simulink model "WindFarmType4AverageModel"  (R2024b)
settings: Solver=FixedStepDiscrete  StartTime=0.0  StopTime=5  RelTol=1e-4
PreLoadFcn:
  | Ts=50e-6;
InitFcn:
  | xInitial = WindFarmType4AverageModelInit;
  | Ts=50e-6;
undefined symbols (not defined in the file or in its folder): D1, D11, Delta, DiscIntNeverNeededParam, find_system
libraries: spsSecondOrderFilterLib x54, spsabctodq0Lib x30, spsThreePhaseVIMeasurementLib x26, simulink_extras x24, spsFirstOrderFilterLib x24, spsControlledVoltageSourceLib x18, spsThreePhaseTransformerTwoWindingsLib x14, spsThreePhasePISectionLineLib x14, simulink x12, spsSeriesRLCBranchLib x7, spsThreePhaseSeriesRLCLoadLib x7, spsSynchronousMachinepuStandardLib x7
(part 1 of 14)
settings Model: Creator=The MathWorks, Inc.  LastModifiedBy=prankfarsons
settings SolverCC: AlgebraicLoopSolver=TrustRegion  SolverResetMethod=Robust
settings DataIOCC: LimitDataPoints=on  SaveFormat=StructureWithTime  SaveOutput=off  SaveTime=off  ReturnWorkspaceOutputs=off
settings OptimizationCC: ExpressionDepthLimit=2147483647  InitFltsAndDblsToZero=on  LifeSpan=inf
settings DebuggingCC: UnderspecifiedInitializationDetection=Classic  MergeDetectMultiDrivingBlocksExec=none  SolverPrmCheckMsg=warning  FcnCallInpInsideContextMsg=warning  UnconnectedInputMsg=warning  UnconnectedOutputMsg=warning  UnconnectedLineMsg=warning  StateNameClashWarn=warning  SubsystemReferenceDiagnosticForUnitTest=warning  SFUnexpectedBacktrackingDiag=warning  SFNoUnconditionalDefaultTransitionDiag=warning  SFExecutionAtInitializationDiag=none  ArithmeticOperatorsInVariantConditions=warning
settings HardwareCC: ProdBitPerPointer=32  ProdBitPerSizeT=32  ProdBitPerPtrDiffT=32  ProdLargestAtomicFloat=None  ProdIntDivRoundTo=Undefined  ProdEndianess=Unspecified  ProdWordSize=32  ProdHWDeviceType=32-bit Generic
settings ModelReferenceCC: EnableRefExpFcnMdlSchedulingChecks=on  PropagateSignalLabelsOutOfModel=off
settings SFSimCC: SimUseLocalCustomCode=off  CustomCodeUndefinedFunction=UseInterfaceOnly
settings RTWCC: RTWUseLocalCustomCode=off  GPUComputeCapability=3.5  DLArmComputeVersion=19.05
settings CodeAppCC: StateflowObjectComments=on
settings GRTTargetCC: TargetLangStandard=C89/C90 (ANSI)  CombineOutputUpdateFcns=off  GRTInterface=on
settings ConfigComp: CovMetricSettings=dw  CovSaveCumulativeToWorkspaceVar=on  CovSaveSingleToWorkspaceVar=on  CovExternalEMLEnable=off  CovSFcnEnable=off
settings SimscapeCC: SimscapeNormalizeSystem=off

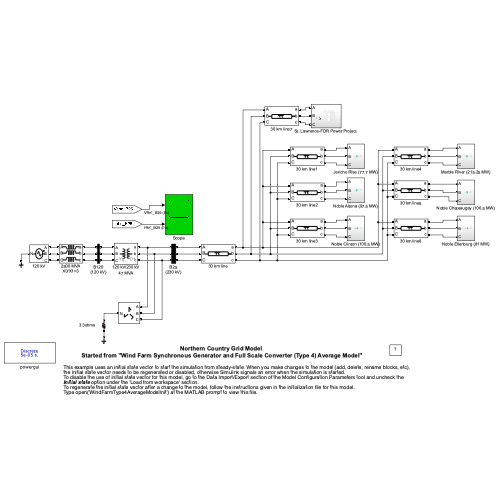
[thumbnail: Simulink's stored preview of the top-level diagram]
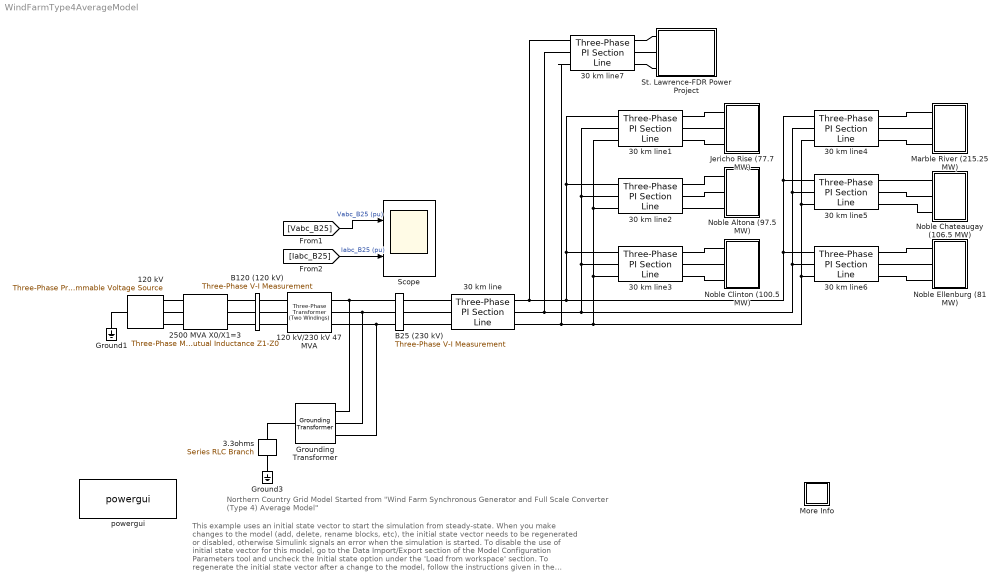
== system WindFarmType4AverageModel ==
  note: Northern Country Grid Model
      | Started from "Wind Farm Synchronous Generator and Full Scale Converter (Type 4) Average Model"
  note: This example uses an initial state vector to start the simulation from steady-state. When you make changes to the model (add, delete, rename blocks, etc),
      | the initial state vector needs to be regenerated or disabled, otherwise Simulink signals an error when the simulation is started.
      | To disable the use of initial state vector for this model, go to the Data Import/Export section of the Model Configuration Parameters tool and uncheck the
      | Initial state option under the 'Load from workspace' section.
      | To regenerate the initial state vector after a change to the model, follow the instructions given in the initialization file for this model.
      | Type open('WindFarmType4AverageModelInit') at the MATLAB prompt to view this file.
  120 kV : spsThreePhaseProgrammableVoltageSourceLib/Three-Phase Programmable Voltage Source  PositiveSequence=[120e3 0 60]  VariationEntity=Amplitude  VariationType=Table of time-amplitude pairs  VariationTypeAlt=Step  VariationStep=-0.2  VariationRate=10  VariationMagnitude=0.3  VariationFrequency=2  VariationTiming=[0.05 0.05+5/60]  VariationPhaseA=off  Amplitudes=[1 0.75 1.0]  TimeValues=[0 0.03 0.13]  HarmonicGeneration=off  HarmonicA=[1 -0.1 0 2]  HarmonicB=[2 0.15 35 2]*0  Timing="[0.1  2]"  BusType=swing  Pref=0  Qref=0  Qmin=-inf  Qmax=inf
  120 kV/230 kV 47 MVA : spsThreePhaseTransformerTwoWindingsLib/Three-Phase Transformer (Two Windings)  Winding1Connection=Yg  Winding2Connection=Delta (D1)  CoreType=Three single-phase transformers  SetSaturation=off  Hysteresis=off  DataFile='basic_model'  SetInitialFlux=off  Measurements=None  UNITS=pu  NominalPower=[47e6 60 ]  Winding1="[ 120e3  0.08/30   0.08 ]"  Winding2="[ 230e3  0.08/30  0.08]"  Rm=500  Lm=500  L0=0.5  Saturation="[ 0,0  ;  0.005,1.2  ;  1.0,1.4 ]"  InitialFluxes=[ 0.8 , -0.8 , 0.7 ]  BreakLoop=off  DiscreteSolver=Trapezoidal iterative  DataType=off  TransfoNumber=0
  2500 MVA X0/X1=3 : spsThreePhaseMutualInductanceZ1Z0Lib/Three-Phase Mutual Inductance Z1-Z0  LConnTagsString=a|b|c  RConnTagsString=A|B|C  PositiveSequence="[0.1  1.0/(2*pi*60)] *120e3^2/2500e6"  ZeroSequence="[0.3  3.0/(2*pi*60)] *120e3^2/2500e6"
      settings: AttributesFormatString=\n
  "3.3ohms " : spsSeriesRLCBranchLib/Series RLC Branch  LConnTagsString=__new0  RConnTagsString=__new0  BranchType=R  Resistance=3.3  Inductance=[]  SetiL0=off  InitialCurrent=0  Capacitance=[]  Setx0=off  InitialVoltage=0  Measurements=None
  30 km line{,1..7} (8 alike) : spsThreePhasePISectionLineLib/Three-Phase PI Section Line  LConnTagsString=a|b|c  RConnTagsString=A|B|C  Length=30  Frequency=60  Resistances=[0.1153 0.413]  Inductances=[1.05e-3 3.32e-3]  Capacitances=[11.33e-009 5.01e-009]
  B120 (120 kV) : spsThreePhaseVIMeasurementLib/Three-Phase V-I Measurement  VoltageMeasurement=no  SetLabelV=off  LabelV=Vabc_B120  Vpu=off  VpuLL=off  CurrentMeasurement=no  SetLabelI=on  LabelI=Iabc_B120  Ipu=off  Pbase=100e6  Vbase=120e3  OutputType=Complex  PhasorSimulation=off  PSBequivalent=0
  B25 (230 kV) : spsThreePhaseVIMeasurementLib/Three-Phase V-I Measurement  VoltageMeasurement=phase-to-ground  SetLabelV=on  LabelV=Vabc_B25  Vpu=on  VpuLL=off  CurrentMeasurement=yes  SetLabelI=on  LabelI=Iabc_B25  Ipu=on  Pbase=77.7e6  Vbase=230e3  OutputType=Complex  PhasorSimulation=off  PSBequivalent=0
  Ground1 : spsGroundLib/Ground  LConnTagsString=a
  Ground3 : spsGroundLib/Ground  LConnTagsString=a
  "Grounding Transformer " : spsGroundingTransformerLib/Grounding Transformer   UNITS=pu  NominalPower="[100e6   60]"  NominalVoltage=25e3  ZeroSequenceImpedance_pu=[0.025 0.75]  MagnetizationBranch_pu=[500 500]  ZeroSequenceImpedance_SI=[0.052083 589.05]  MagnetizationBranch_SI=[1041.7 3.927e+005]  Measurements=None
  Jericho Rise (77.7 MW) : Subsystem
  Marble River (215.25 MW) : Subsystem
  More Info : Subsystem
      settings: OpenFcn="showExample(\"simscapeelectricalsps/WindFarmType4AverageModelExample\")"
      mask Display: disp('?')
  Noble Altona (97.5 MW) : Subsystem
  Noble Chateaugay (106.5 MW) : Subsystem
  Noble Clinton (100.5 MW) : Subsystem
  Noble Ellenburg (81 MW) : Subsystem
  Scope : Scope  NumInputPorts=2
  "St. Lawrence-FDR Power Project " : Subsystem
  powergui : spspowerguiLib/powergui  SimulationMode=Discrete  SampleTime=Ts  frequency=60  Iterations=50  frequencyindice=0  Pbase=100e6  ErrMax=1e-4  UnitsV=kV  UnitsW=MW  buscounter=0  FunctionMessages=off  echomessages=off  EnableUseOfTLC=off  CurrentSourceSwitches=off  DisableSnubberDevices=off  DisableRonSwitches=off  DisableVfSwitches=off  DisplayEquations=off  AutomaticDiscreteSolvers=off  SolverType=Tustin/Backward Euler (TBE)  Interpol=off  ExternalGateDelay=off  methode=off  Ts=0  x0status=blocks  SPID=off  SwTol=0  HookPort=off  NonlinearTolerance=1e-4  nMaxIteration=100  ContinueOnMaxIteration=off  RestoreLinks=warning  ResistiveCurrentMeasurement=off  Frange=[0:2:500]  Ylog=off  Xlog=on  ShowGrid=off  save=off  variable=ZData  structure=0  ZoomFFT=on  StartTime=0.0  cycles=1  DisplayStyle=1  fundamental=60  FreqAxis=off  MaxFrequency=1000  frequencyindicesteady=1  RmsSteady=1  display=off
  wires:
  [Vabc_B25] -> Scope/1  "Vabc_B25 (pu)"
  [Iabc_B25] -> Scope/2  "Iabc_B25 (pu)"
  connections:
  B25 (230 kV)/LConn2 -- 120 kV/230 kV 47 MVA/RConn2 -- "Grounding Transformer "/LConn2
  B25 (230 kV)/LConn3 -- 120 kV/230 kV 47 MVA/RConn3 -- "Grounding Transformer "/LConn3
  B25 (230 kV)/LConn1 -- 120 kV/230 kV 47 MVA/RConn1 -- "Grounding Transformer "/LConn1
  "3.3ohms "/RConn1 -- Ground3/LConn1
  2500 MVA X0/X1=3/RConn1 -- B120 (120 kV)/LConn1
  2500 MVA X0/X1=3/RConn2 -- B120 (120 kV)/LConn2
  2500 MVA X0/X1=3/RConn3 -- B120 (120 kV)/LConn3
  B120 (120 kV)/RConn1 -- 120 kV/230 kV 47 MVA/LConn1
  B120 (120 kV)/RConn2 -- 120 kV/230 kV 47 MVA/LConn2
  B120 (120 kV)/RConn3 -- 120 kV/230 kV 47 MVA/LConn3
  30 km line/LConn1 -- B25 (230 kV)/RConn1
  30 km line/LConn2 -- B25 (230 kV)/RConn2
  30 km line/LConn3 -- B25 (230 kV)/RConn3
  "3.3ohms "/LConn1 -- "Grounding Transformer "/RConn1
  Ground1/LConn1 -- 120 kV/LConn1
  2500 MVA X0/X1=3/LConn1 -- 120 kV/RConn1
  2500 MVA X0/X1=3/LConn2 -- 120 kV/RConn2
  2500 MVA X0/X1=3/LConn3 -- 120 kV/RConn3
  30 km line4/RConn1 -- Marble River (215.25 MW)/LConn1
  30 km line4/RConn2 -- Marble River (215.25 MW)/LConn2
  30 km line4/RConn3 -- Marble River (215.25 MW)/LConn3
  30 km line5/RConn1 -- Noble Chateaugay (106.5 MW)/LConn1
  30 km line5/RConn2 -- Noble Chateaugay (106.5 MW)/LConn2
  30 km line5/RConn3 -- Noble Chateaugay (106.5 MW)/LConn3
  30 km line6/RConn1 -- Noble Ellenburg (81 MW)/LConn1
  30 km line6/RConn2 -- Noble Ellenburg (81 MW)/LConn2
  30 km line6/RConn3 -- Noble Ellenburg (81 MW)/LConn3
  30 km line1/RConn1 -- Jericho Rise (77.7 MW)/LConn1
  30 km line1/RConn2 -- Jericho Rise (77.7 MW)/LConn2
  30 km line1/RConn3 -- Jericho Rise (77.7 MW)/LConn3
  30 km line2/RConn1 -- Noble Altona (97.5 MW)/LConn1
  30 km line2/RConn2 -- Noble Altona (97.5 MW)/LConn2
  30 km line2/RConn3 -- Noble Altona (97.5 MW)/LConn3
  30 km line3/RConn1 -- Noble Clinton (100.5 MW)/LConn1
  30 km line3/RConn2 -- Noble Clinton (100.5 MW)/LConn2
  30 km line3/RConn3 -- Noble Clinton (100.5 MW)/LConn3
  30 km line1/LConn1 -- 30 km line2/LConn1 -- 30 km line3/LConn1 -- 30 km line6/LConn1 -- 30 km line5/LConn1 -- 30 km line4/LConn1 -- 30 km line7/LConn1 -- 30 km line/RConn1
  30 km line1/LConn2 -- 30 km line2/LConn2 -- 30 km line3/LConn2 -- 30 km line6/LConn2 -- 30 km line5/LConn2 -- 30 km line4/LConn2 -- 30 km line7/LConn2 -- 30 km line/RConn2
  30 km line1/LConn3 -- 30 km line2/LConn3 -- 30 km line6/LConn3 -- 30 km line5/LConn3 -- 30 km line4/LConn3 -- 30 km line7/LConn3 -- 30 km line/RConn3 -- 30 km line3/LConn3
  30 km line7/RConn1 -- "St. Lawrence-FDR Power Project "/LConn1
  30 km line7/RConn2 -- "St. Lawrence-FDR Power Project "/LConn2
  30 km line7/RConn3 -- "St. Lawrence-FDR Power Project "/LConn3

== system WindFarmType4AverageModel/Jericho Rise (77.7 MW) ==
  230 kV/34.5 kV 47 MVA : spsThreePhaseTransformerTwoWindingsLib/Three-Phase Transformer (Two Windings)  Winding1Connection=Yg  Winding2Connection=Delta (D1)  CoreType=Three single-phase transformers  SetSaturation=off  Hysteresis=off  DataFile='basic_model'  SetInitialFlux=off  Measurements=None  UNITS=pu  NominalPower=[47e6 60 ]  Winding1="[ 230e3  0.08/30   0.08 ]"  Winding2="[34.5e3  0.08/30  0.08]"  Rm=500  Lm=500  L0=0.5  Saturation="[ 0,0  ;  0.005,1.2  ;  1.0,1.4 ]"  InitialFluxes=[ 0.8 , -0.8 , 0.7 ]  BreakLoop=off  DiscreteSolver=Trapezoidal iterative  DataType=off  TransfoNumber=0
  34.5 kV/ 690V 5*2.5 MVA : spsThreePhaseTransformerTwoWindingsLib/Three-Phase Transformer (Two Windings)  Winding1Connection=Delta (D11)  Winding2Connection=Yg  CoreType=Three single-phase transformers  SetSaturation=off  Hysteresis=off  DataFile='hysteresis'  SetInitialFlux=off  Measurements=None  UNITS=pu  NominalPower="[2.5e6*5  60]"  Winding1=[34.5e3 , 0.025/30 , 0.025]  Winding2=[690, 0.025/30 , 0.025]  Rm=500  Lm=inf  L0=0.5  Saturation=[ 0,0 ; 0.0024,1.2 ; 1.0,1.52 ]  InitialFluxes=[ 0.8 , -0.8 , 0.7 ]  BreakLoop=off  DiscreteSolver=Trapezoidal iterative  DataType=off  TransfoNumber=0
  5 km line : spsThreePhasePISectionLineLib/Three-Phase PI Section Line  LConnTagsString=a|b|c  RConnTagsString=A|B|C  Length=5  Frequency=60  Resistances=[0.1153 0.413]  Inductances=[1.05e-3 3.32e-3]  Capacitances=[11.33e-009 5.01e-009]
  B1 (690 V) : spsThreePhaseVIMeasurementLib/Three-Phase V-I Measurement  VoltageMeasurement=phase-to-ground  SetLabelV=on  LabelV=Vabc_B1  Vpu=on  VpuLL=off  CurrentMeasurement=yes  SetLabelI=on  LabelI=Iabc_B1  Ipu=on  Pbase=37*2.1e6/0.9  Vbase=690  OutputType=Complex  PhasorSimulation=off  PSBequivalent=0
  Bus Selector : BusSelector  OutputSignals=Vdc_V,wr_pu,PQ_pu.P_pu,PQ_pu.Q_pu
  Constant : Constant  Value=15
  Constant1 : Constant  Value=0
  Demux : Demux  Outputs=2
  MW : Gain  Gain=37*2.1/0.9  SaturateOnIntegerOverflow=on  OutDataTypeStr=Inherit: Same as input  ParamDataTypeStr=Inherit: Same as input
  Mux : Mux  Inputs=2
  Wind Farm : Subsystem  LoadFcn=%find_system(gcs,'FollowLinks', 'on', 'LookUnderMasks', 'all');  mask(Wind Turbine: Model 7){Nb_wt=37, ShowParameters=Generator data for 1 wind turbine, nom=[2.1e6/0.9 690 60], Reactances=[ 1.305, 0.296, 0.252, 0.474,  0.243,  0.18 ], Time_constants=[  4.49  0.0681  0.0513  ], Resistance=0.006, mec=[0.62 0.01 1], init=[ 0  0  0  0  0  0  0  0  1 ], Vnom=575, Imax_grid_conv=1.1, RL_grid=[ 0.15 0.15/50], C_var_filter1=150e3, Vdc_nom=1100, C_DClink1=90000e-6, L_R_Boost=[0.0012     5e-3], Pmec1=2e6, wind_speed_CpMax=11, wind0=11, DisplayTurbChar=off, H_WT=4.32, Ksh=0.3, D_mutual=1.5, w_wt0=1, torque0=1, Kdc=[1.1   27.5], Ki_var_reg=0.05, Ki_volt_reg=2, Kgrid_side_cur_reg=[1  50], Kspeed=[5 1], Kboost_cur_reg=[0.025 100], Kp_pitch=15, Kcompensation=[1.5  6], Kfield=[10  20], pitch_max=27, pitch_rate=10, Ts=Ts}
      mask prompts: Nb_wt "Number of wind turbines:"; ShowParameters "Display:"; nom "Nom. power, L-L volt. and freq.: [Pn (VA), Vn (Vrms), fn (Hz)]"; Reactances "Reactances [Xd Xd' Xd'' Xq Xq'' Xl] (p.u.):"; Time_constants "Time constants [Tdo' Tdo'' Tq''] (s):"; Resistance "Resistance Rs (p.u.):"; mec "Inertia constant, friction factor, and pairs of poles: [ H(s)  F(p.u.)  p ]"; init "Initial conditions: [dw(%) th(deg) ia,ib,ic(pu) pha,phb,phc(deg) Vf(pu)]:"; Vnom "Grid-side converter nominal AC voltage (V):"; Imax_grid_conv "Grid-side converter maximum AC current (pu based on generator power and converter nominal AC voltage):"; RL_grid "Grid-side coupling inductor [ L(pu) R(pu),pu based on generator power and converter nominal AC voltage] :"; C_var_filter1 "Line filter capacitor (Q=50) (var):"; Vdc_nom "Nominal DC bus voltage (V)"; C_DClink1 "DC bus capacitor (F):"; L_R_Boost "Boost converter inductance [L(H) R(ohm)]:"; Pmec1 "Nominal mechanical output power (W):"; wind_speed_CpMax "Wind speed at nominal speed and at Cp max (must be between 6 m/s and 30 m/s) (m/s):"; wind0 "Initial wind speed (m/s):"; DisplayTurbChar "Display wind turbine power characteristics:"; H_WT "Wind turbine inertia constant H (s):"; Ksh "Shaft spring constant refer to high-speed shaft (pu of nominal mechanical torque/rad):"; D_mutual "Shaft mutual damping (pu of nominal mechanical torque/pu dw):"; w_wt0 "Turbine initial speed (pu of nominal speed):"; torque0 "Initial output torque (pu of nominal mechanical torque):"; Kdc "DC bus voltage regulator gains [Kp Ki]:"; Ki_var_reg "Grid-side converter var regulator gain [ Ki]:"; Ki_volt_reg "Grid-side converter voltage regulator gain [ Ki]:"; Kgrid_side_cur_reg "Grid-side converter current regulator gains [Kp Ki]:"; Kspeed "Speed regulator gains [Kp Ki]:"; Kboost_cur_reg "Boost inductor current regulator gains [Kp Ki]:"; Kp_pitch "Pitch controller gain [Kp]:"; Kcompensation "Pitch compensation gains [Kp Ki]:"; Kfield "Field excitation gains [Kp Ki]:"; pitch_max "Maximum pitch angle (deg):"; pitch_rate "Maximum rate of change of pitch angle (deg/s)"; Ts "Sample time (s):"
      mask help: This block implements a model of a variable speed pitch controlled wind turbine using a synchronous generator.
      mask init:
      | %Generator data
      | Pnom=nom(1)*Nb_wt;
      | Vnom_gen=nom(2);
      | Fnom=nom(3);
      | Xd=Reactances(1);
      | Xd1=Reactances(2);
      | Xd2=Reactances(3);
      | Xq=Reactances(4);
      | Xq2=Reactances(5);
      | Xl=Reactances(6);
      | Tdo1=Time_constants(1);
      | Tdo2=Time_constants(2);
      | Tq2=Time_constants(3);
      | H=mec(1);
      | F=mec(2);
      | p=mec(3);
      | 
      | % Converters data
      | L_RL=RL_grid(1);
      | R_RL=RL_grid(2);
      | L_Boost=L_R_Boost(1)/Nb_wt;
      | R_Boost=L_R_Boost(2)/Nb_wt;
      | Q_filter=50;
      | C_DClink=C_DClink1*Nb_wt;
      | C_var_filter=C_var_filter1*Nb_wt;
      | 
      | % Controller data
      | Freq_filter=10000;   %Hz
      | Zeta_filter=0.707;
      | Kp_dc=Kdc(1);
      | Ki_dc=Kdc(2);
      | Kp_grid_side_cur_reg=Kgrid_side_cur_reg(1);
      | Ki_grid_side_cur_reg=Kgrid_side_cur_reg(2);
      | Kp_speed=Kspeed(1);
      | Ki_speed=Kspeed(2);
      | Kp_boost_cur_reg=Kboost_cur_reg(1);
      | Ki_boost_cur_reg=Kboost_cur_reg(2);
      | Kp_compensation=Kcompensation(1);
      | Ki_compensation=Kcompensation(2);
      | Kp_field=Kfield(1);
      | Ki_field=Kfield(2);
      | Mod_index_max=1.1;
      | T_speed=5;      %Speed reference time constant (s)
      | Iq_ref_limit_time_constant=0.3; %(s)
      | Current_reg_output_limit=1.1;   %(pu)
      | Var_reg_output_hi_limit=1.1;    %(pu)
      | Var_reg_output_low_limit=0.9;   %(pu)
      | Pitch_time_constant=0.01;       %(s)
      | Vf_limit=10;    %Field voltage limit (pu)
      | Flux_meas_time_constant=1*(1/Fnom); %(s)
      | Ts_snub=50e-6;  %Sample time to compute snubber resistance
      | 
      | 
      | % Turbine data
      | Pmec=Pmec1*Nb_wt;
      | c1 = 0.6450;
      | c2 = 116;
      | c3 = .4;
      | c4 = 5;
      | c5 = 21;
      | c6 = .00912;  % Set Pmin in stall condition (does not vary with wind_speed_Pmax)
      | c7 = .08;
      | c8 = .035;
      | theta=0;
      | CpMax=.5;
      | lambda_CpMax=9.9495;
      | 
      | c1_c8=[c1 c2 c3 c4 c5 c6 c7 c8];
      |   
      | 
      | %   Cp = c1*(c6*lambda + (-c4 - c3*(2.5 + theta) + c2*(1/(lambda + ...
      | %   c7*(2.5 + theta)) - c8/(1 + (2.5 + theta)^3)))/exp(c5*(1/(lambda + ...
      | %   c7*(2.5 + theta)) - c8/(1 + (2.5 + theta)^3))))
      | 
      | 
      |         %%%%%%%%%%%%%%%%%%%%%%%%%%%%%%%%%%%%%%%%%%%%%%%%%%%%%%%%%%%%%%%%%%%%%%%%%%%
      |         % Operation at Cp max
      |         %%%%%%%%%%%%%%%%%%%%%%%%%%%%%%%%%%%%%%%%%%%%%%%%%%%%%%%%%%%%%%%%%%%%%%%%%%%
      |         
      |         rated_omegar=1;
      |         omegar = rated_omegar;
      |         
      |         % Enforce boundaries on wind speed
      |         % A warning could be displayed
      |         if wind_speed_CpMax < 6
      |             wind_speed_CpMax=6;
      |             disp('Warning: Wind speed at nominal speed and at Cp max has been set to 6 m/s')
      |         end
      |         if wind_speed_CpMax > 30
      |             wind_speed_CpMax=30;
      |             disp('Warning: Wind speed at nominal speed and at Cp max has been set to 30 m/s')
      |         end
      | 
      |         K1=lambda_CpMax/omegar*wind_speed_CpMax;
      |         
      |         % Calculation of K2 needed to get P equal to the requested value at
      |         % Cp max for the requested wind speed
      |         
      |         Prated=Pmec;
      |         P_rated_omegar_theta_zero=0.75;
      |         
      |         K2 = P_rated_omegar_theta_zero*Prated/(wind_speed_CpMax^3*CpMax);
      |         
      |         K1_K2=[K1 K2];
      |         
      |         %%%%%%%%%%%%%%%%%%%%%%%%%%%%%%%%%%%%%%%%%%%%%%%%%%%%%%%%%%%%%%%%%%%%%%%%%%%
      |         % End of calculation for operation at Cp max
      |         %%%%%%%%%%%%%%%%%%%%%%%%%%%%%%%%%%%%%%%%%%%%%%%%%%%%%%%%%%%%%%%%%%%%%%%%%%%
      |         
      | 
      | %%%%%%%%%%%%%%%%%%%%%%%%%%%%%%%%%%%%%%%%%%%%%%%%%%%%%%%%%%%%%%%%%%%%%%%%%%%
      | % Plot turbine characteristics
      | %%%%%%%%%%%%%%%%%%%%%%%%%%%%%%%%%%%%%%%%%%%%%%%%%%%%%%%%%%%%%%%%%%%%%%%%%%% 
      | 
      | DisplayTurbChar=get_param(gcb,'DisplayTurbChar');
      | if strcmp(DisplayTurbChar,'on')
      |     vect_theta = 0:2:30;
      |     
      |     vect_lambda = 1:0.2:30;
      |     
      |     clear Cp;
      |     
      |     for i=1:length(vect_theta)
      |      for j=1:length(vect_lambda)
      |                 Cp(i,j) = c1*(c6*vect_lambda(j) + (-c4 - c3*(2.5 + vect_theta(i)) + c2*(1/(vect_lambda(j) + ...
      |                 c7*(2.5 + vect_theta(i))) - c8/(1 + (2.5 + vect_theta(i))^3)))/exp(c5*(1/(vect_lambda(j) + ...
      |                 c7*(2.5 + vect_theta(i))) - c8/(1 + (2.5 + vect_theta(i))^3))));
      |      end
      |     end
      | 
      |     figure(1);
      |     clf;
      |     hold on;
      | 
      |     plot(vect_lambda, Cp);
      |     axis([0, 25, 0, .6]);
      |     title('Wind Turbine Cp Characteristic (pitch angle increases by step of 2 deg.)');
      |     ylabel('Cp');
      |     set(gca,'ytick',[0 .1 .2 .3 .4 .5 .6]);
      |     xlabel('Lambda');
      |     grid on;
      |     text(10.1,0.51,'Pitch angle 0 degree');
      | 
      |     hold off
      |     
      |     % Plot of the wind turbine mechanical power output (pu) lambda and Cp
      |     % characteristics against wind speed (m/s) for a range of theta.
      |     
      |     wind_speed_range = [1,.2,30];
      |     vect_wind_speed = 1:0.2:30;
      |     
      |     clear lambda;
      |     clear Cp;
      |     clear P;
      | 
      |     for i=1:length(vect_theta)
      |         for j=1:length(vect_wind_speed)
      |             lambda(i,j) = K1*omegar/vect_wind_speed(j);
      |             Cp(i,j) = c1*(c6*lambda(i,j) + (-c4 - c3*(2.5 + vect_theta(i)) + c2*(1/(lambda(i,j) + ...
      |             c7*(2.5 + vect_theta(i))) - c8/(1 + (2.5 + vect_theta(i))^3)))/exp(c5*(1/(lambda(i,j) + ...
      |             c7*(2.5 + vect_theta(i))) - c8/(1 + (2.5 + vect_theta(i))^3))));
      |             P(i,j) = K2/Prated*vect_wind_speed(j)^3*Cp(i,j);
      |         end
      |     end
      |     
      |     
      |     figure(2);
      |     clf;
      |     hold on
      |     
      |     subplot(3,1,1);
      |     plot(vect_wind_speed, P);
      |     axis([0, 35, 0, 1.5]);
      |     title('Wind Turbine Characteristics (w = 1 pu, pitch angle increases by step of 2 deg.)');
      |     ylabel('P (pu)');
      |     set(gca,'ytick',0:.5:4);
      |     grid on;
      |     
      |     subplot(3,1,2);
      |     plot(vect_wind_speed, lambda);
      |     axis([0, 35, 0, 20]);
      |     ylabel('Lambda');
      |     grid on;
      |     
      |     subplot(3,1,3)
      |     plot(vect_wind_speed, Cp);
      |     axis([0, 35, 0, .6]);
      |     xlabel('Wind Speed (m/s)');
      |     ylabel('Cp');
      |     set(gca,'ytick',[0 .1 .2 .3 .4 .5 .6]);
      |     grid on;
      | 
      |     hold off
      |     set_param(gcb,'DisplayTurbChar','off')
      |     
      | end
      mask TypeOptions ShowParameters: Generator data for 1 wind turbine | Converters data for 1 wind turbine | Turbine data for 1 wind turbine | Drive train data for 1 wind turbine | Control parameters for 1 wind turbine
      mask Callback ShowParameters:
      | BlockName=getfullname(gcb);
      | %
      | Param_Show=get_param(BlockName,'ShowParameters');
      | Param_DisplayTurbChar=get_param(BlockName,'DisplayTurbChar');
      | 
      | p_mask{3}='off';p_mask{4}='off';p_mask{5}='off';
      | p_mask{6}='off';p_mask{7}='off';p_mask{8}='off';p_mask{9}='off';
      | p_mask{10}='off';p_mask{11}='off';p_mask{12}='off';p_mask{13}='off';
      | p_mask{14}='off';p_mask{15}='off';p_mask{16}='off';p_mask{17}='off';
      | p_mask{18}='off';p_mask{19}='off';p_mask{20}='off';p_mask{21}='off';
      | p_mask{22}='off';p_mask{23}='off';p_mask{24}='off';p_mask{25}='off';
      | p_mask{26}='off';p_mask{27}='off';p_mask{28}='off';p_mask{29}='off';
      | p_mask{30}='off';p_mask{31}='off';p_mask{32}='off';p_mask{33}='off';
      | p_mask{34}='off';p_mask{35}='off';
      | 
      | switch Param_Show
      | 	case 'Generator data for 1 wind turbine'
      | 		p_mask{3}='on';p_mask{4}='on';p_mask{5}='on';
      |         p_mask{6}='on';p_mask{7}='on';p_mask{8}='on';
      |     case 'Converters data for 1 wind turbine'
      | 		p_mask{9}='on';p_mask{10}='on';p_mask{11}='on';
      |         p_mask{12}='on';p_mask{13}='on';p_mask{14}='on';p_mask{15}='on';
      | 	case 'Turbine data for 1 wind turbine'
      | 		p_mask{16}='on';p_mask{17}='on';p_mask{18}='on';p_mask{19}='on';
      |     case 'Drive train data for 1 wind turbine'
      |         p_mask{20}='on';p_mask{21}='on';p_mask{22}='on';p_mask{23}='on';
      |         p_mask{24}='on';
      |     case 'Control parameters for 1 wind turbine'
      |         p_mask{25}='on';p_mask{26}='on';p_mask{27}='on';
      |         p_mask{28}='on';p_mask{29}='on';p_mask{30}='on';p_mask{31}='on';
      |         p_mask{32}='on';p_mask{33}='on';p_mask{34}='on';p_mask{35}='on';
      | end
      | 
      | ParVisible={'on','on',p_mask{3},p_mask{4},p_mask{5},p_mask{6},...
      |     p_mask{7},p_mask{8},p_mask{9},p_mask{10},p_mask{11},p_mask{12},...
      |     p_mask{13},p_mask{14},p_mask{15},p_mask{16},p_mask{17},p_mask{18},...
      |     p_mask{19},p_mask{20},p_mask{21},p_mask{22},p_mask{23},p_mask{24},...
      |     p_mask{25},p_mask{26},p_mask{27},p_mask{28},p_mask{29},p_mask{30},...
      |     p_mask{31},p_mask{32},p_mask{33},p_mask{34},p_mask{35},'on'};
      | %
      | set_param(BlockName,'MaskVisibilities',ParVisible);
      | set_param(BlockName,'DisplayTurbChar',Param_DisplayTurbChar);
      mask Display: disp(' ');
  Wind Farm Scope : Scope  NumInputPorts=6
  A : PMIOPort  Side=Left
  B : PMIOPort  Port=2  Side=Left
  C : PMIOPort  Port=3  Side=Left
  wires:
  Constant1/1 -> Wind Farm/2(Qref_pu)
  [Vabc_B1] -> Wind Farm Scope/1  "Vabc_B575 (pu)"
  Demux/1 -> Wind Farm Scope/5  "P (MW)"
  Bus Selector/1 -> Wind Farm Scope/3  "<Vdc_V>"
  Demux/2 -> Wind Farm Scope/6  "Q (Mvar)"
  Mux/1 -> MW/1
  Bus Selector/2 -> Wind Farm Scope/4  "<wr_pu>"
  Wind Farm/1(m) -> Bus Selector/1
  Bus Selector/3 -> Mux/1  "<P_pu>"
  Bus Selector/4 -> Mux/2  "<Q_pu>"
  MW/1 -> Demux/1
  [Iabc_B1] -> Wind Farm Scope/2  "Iabc_B575 (pu)"
  Constant/1 -> Wind Farm/1("Wind (m/s) ")
  connections:
  B1 (690 V)/LConn2 -- 34.5 kV/ 690V 5*2.5 MVA/RConn2
  B1 (690 V)/RConn1 -- Wind Farm/LConn1
  B1 (690 V)/LConn1 -- 34.5 kV/ 690V 5*2.5 MVA/RConn1
  B1 (690 V)/LConn3 -- 34.5 kV/ 690V 5*2.5 MVA/RConn3
  B1 (690 V)/RConn3 -- Wind Farm/LConn3
  Wind Farm/LConn2 -- B1 (690 V)/RConn2
  5 km line/RConn1 -- 34.5 kV/ 690V 5*2.5 MVA/LConn1
  5 km line/RConn2 -- 34.5 kV/ 690V 5*2.5 MVA/LConn2
  5 km line/LConn1 -- 230 kV/34.5 kV 47 MVA/RConn1
  5 km line/LConn2 -- 230 kV/34.5 kV 47 MVA/RConn2
  5 km line/LConn3 -- 230 kV/34.5 kV 47 MVA/RConn3
  A/RConn1 -- 230 kV/34.5 kV 47 MVA/LConn1
  B/RConn1 -- 230 kV/34.5 kV 47 MVA/LConn2
  C/RConn1 -- 230 kV/34.5 kV 47 MVA/LConn3
  5 km line/RConn3 -- 34.5 kV/ 690V 5*2.5 MVA/LConn3

== system WindFarmType4AverageModel/Marble River (215.25 MW) ==
  230 kV/34.5 kV 47 MVA : spsThreePhaseTransformerTwoWindingsLib/Three-Phase Transformer (Two Windings)  Winding1Connection=Yg  Winding2Connection=Delta (D1)  CoreType=Three single-phase transformers  SetSaturation=off  Hysteresis=off  DataFile='basic_model'  SetInitialFlux=off  Measurements=None  UNITS=pu  NominalPower=[47e6 60 ]  Winding1="[ 230e3  0.08/30   0.08 ]"  Winding2="[34.5e3  0.08/30  0.08]"  Rm=500  Lm=500  L0=0.5  Saturation="[ 0,0  ;  0.005,1.2  ;  1.0,1.4 ]"  InitialFluxes=[ 0.8 , -0.8 , 0.7 ]  BreakLoop=off  DiscreteSolver=Trapezoidal iterative  DataType=off  TransfoNumber=0
  34.5 kV/ 690V 5*2.5 MVA : spsThreePhaseTransformerTwoWindingsLib/Three-Phase Transformer (Two Windings)  Winding1Connection=Delta (D11)  Winding2Connection=Yg  CoreType=Three single-phase transformers  SetSaturation=off  Hysteresis=off  DataFile='hysteresis'  SetInitialFlux=off  Measurements=None  UNITS=pu  NominalPower="[2.5e6*5  60]"  Winding1=[34.5e3 , 0.025/30 , 0.025]  Winding2=[690, 0.025/30 , 0.025]  Rm=500  Lm=inf  L0=0.5  Saturation=[ 0,0 ; 0.0024,1.2 ; 1.0,1.52 ]  InitialFluxes=[ 0.8 , -0.8 , 0.7 ]  BreakLoop=off  DiscreteSolver=Trapezoidal iterative  DataType=off  TransfoNumber=0
  5 km line : spsThreePhasePISectionLineLib/Three-Phase PI Section Line  LConnTagsString=a|b|c  RConnTagsString=A|B|C  Length=5  Frequency=60  Resistances=[0.1153 0.413]  Inductances=[1.05e-3 3.32e-3]  Capacitances=[11.33e-009 5.01e-009]
  B2 (690 V) : spsThreePhaseVIMeasurementLib/Three-Phase V-I Measurement  VoltageMeasurement=phase-to-ground  SetLabelV=on  LabelV=Vabc_B2  Vpu=on  VpuLL=off  CurrentMeasurement=yes  SetLabelI=on  LabelI=Iabc_B2  Ipu=on  Pbase=5*2e6/0.9  Vbase=690  OutputType=Complex  PhasorSimulation=off  PSBequivalent=0
  Bus Selector : BusSelector  OutputSignals=Vdc_V,wr_pu,PQ_pu.P_pu,PQ_pu.Q_pu
  Constant : Constant  Value=15
  Constant1 : Constant  Value=0
  Demux : Demux  Outputs=2
  MW : Gain  Gain=70*3.075/0.9  SaturateOnIntegerOverflow=on  OutDataTypeStr=Inherit: Same as input  ParamDataTypeStr=Inherit: Same as input
  Mux : Mux  Inputs=2
  Wind Farm : Subsystem  LoadFcn=%find_system(gcs,'FollowLinks', 'on', 'LookUnderMasks', 'all');  mask(Wind Turbine: Model 7){Nb_wt=70, ShowParameters=Generator data for 1 wind turbine, nom=[3.075e6/0.9 690 60], Reactances=[ 1.305, 0.296, 0.252, 0.474,  0.243,  0.18 ], Time_constants=[  4.49  0.0681  0.0513  ], Resistance=0.006, mec=[0.62 0.01 1], init=[ 0  0  0  0  0  0  0  0  1 ], Vnom=575, Imax_grid_conv=1.1, RL_grid=[ 0.15 0.15/50], C_var_filter1=150e3, Vdc_nom=1100, C_DClink1=90000e-6, L_R_Boost=[0.0012     5e-3], Pmec1=2e6, wind_speed_CpMax=11, wind0=11, DisplayTurbChar=off, H_WT=4.32, Ksh=0.3, D_mutual=1.5, w_wt0=1, torque0=1, Kdc=[1.1   27.5], Ki_var_reg=0.05, Ki_volt_reg=2, Kgrid_side_cur_reg=[1  50], Kspeed=[5 1], Kboost_cur_reg=[0.025 100], Kp_pitch=15, Kcompensation=[1.5  6], Kfield=[10  20], pitch_max=27, pitch_rate=10, Ts=Ts}
      mask prompts: Nb_wt "Number of wind turbines:"; ShowParameters "Display:"; nom "Nom. power, L-L volt. and freq.: [Pn (VA), Vn (Vrms), fn (Hz)]"; Reactances "Reactances [Xd Xd' Xd'' Xq Xq'' Xl] (p.u.):"; Time_constants "Time constants [Tdo' Tdo'' Tq''] (s):"; Resistance "Resistance Rs (p.u.):"; mec "Inertia constant, friction factor, and pairs of poles: [ H(s)  F(p.u.)  p ]"; init "Initial conditions: [dw(%) th(deg) ia,ib,ic(pu) pha,phb,phc(deg) Vf(pu)]:"; Vnom "Grid-side converter nominal AC voltage (V):"; Imax_grid_conv "Grid-side converter maximum AC current (pu based on generator power and converter nominal AC voltage):"; RL_grid "Grid-side coupling inductor [ L(pu) R(pu),pu based on generator power and converter nominal AC voltage] :"; C_var_filter1 "Line filter capacitor (Q=50) (var):"; Vdc_nom "Nominal DC bus voltage (V)"; C_DClink1 "DC bus capacitor (F):"; L_R_Boost "Boost converter inductance [L(H) R(ohm)]:"; Pmec1 "Nominal mechanical output power (W):"; wind_speed_CpMax "Wind speed at nominal speed and at Cp max (must be between 6 m/s and 30 m/s) (m/s):"; wind0 "Initial wind speed (m/s):"; DisplayTurbChar "Display wind turbine power characteristics:"; H_WT "Wind turbine inertia constant H (s):"; Ksh "Shaft spring constant refer to high-speed shaft (pu of nominal mechanical torque/rad):"; D_mutual "Shaft mutual damping (pu of nominal mechanical torque/pu dw):"; w_wt0 "Turbine initial speed (pu of nominal speed):"; torque0 "Initial output torque (pu of nominal mechanical torque):"; Kdc "DC bus voltage regulator gains [Kp Ki]:"; Ki_var_reg "Grid-side converter var regulator gain [ Ki]:"; Ki_volt_reg "Grid-side converter voltage regulator gain [ Ki]:"; Kgrid_side_cur_reg "Grid-side converter current regulator gains [Kp Ki]:"; Kspeed "Speed regulator gains [Kp Ki]:"; Kboost_cur_reg "Boost inductor current regulator gains [Kp Ki]:"; Kp_pitch "Pitch controller gain [Kp]:"; Kcompensation "Pitch compensation gains [Kp Ki]:"; Kfield "Field excitation gains [Kp Ki]:"; pitch_max "Maximum pitch angle (deg):"; pitch_rate "Maximum rate of change of pitch angle (deg/s)"; Ts "Sample time (s):"
      mask help: This block implements a model of a variable speed pitch controlled wind turbine using a synchronous generator.
      mask init: same as WindFarmType4AverageModel/Jericho Rise (77.7 MW)/Wind Farm
      mask TypeOptions ShowParameters: Generator data for 1 wind turbine | Converters data for 1 wind turbine | Turbine data for 1 wind turbine | Drive train data for 1 wind turbine | Control parameters for 1 wind turbine
      mask Callback ShowParameters:
      | BlockName=getfullname(gcb);
      | %
      | Param_Show=get_param(BlockName,'ShowParameters');
      | Param_DisplayTurbChar=get_param(BlockName,'DisplayTurbChar');
      | 
      | p_mask{3}='off';p_mask{4}='off';p_mask{5}='off';
      | p_mask{6}='off';p_mask{7}='off';p_mask{8}='off';p_mask{9}='off';
      | p_mask{10}='off';p_mask{11}='off';p_mask{12}='off';p_mask{13}='off';
      | p_mask{14}='off';p_mask{15}='off';p_mask{16}='off';p_mask{17}='off';
      | p_mask{18}='off';p_mask{19}='off';p_mask{20}='off';p_mask{21}='off';
      | p_mask{22}='off';p_mask{23}='off';p_mask{24}='off';p_mask{25}='off';
      | p_mask{26}='off';p_mask{27}='off';p_mask{28}='off';p_mask{29}='off';
      | p_mask{30}='off';p_mask{31}='off';p_mask{32}='off';p_mask{33}='off';
      | p_mask{34}='off';p_mask{35}='off';
      | 
      | switch Param_Show
      | 	case 'Generator data for 1 wind turbine'
      | 		p_mask{3}='on';p_mask{4}='on';p_mask{5}='on';
      |         p_mask{6}='on';p_mask{7}='on';p_mask{8}='on';
      |     case 'Converters data for 1 wind turbine'
      | 		p_mask{9}='on';p_mask{10}='on';p_mask{11}='on';
      |         p_mask{12}='on';p_mask{13}='on';p_mask{14}='on';p_mask{15}='on';
      | 	case 'Turbine data for 1 wind turbine'
      | 		p_mask{16}='on';p_mask{17}='on';p_mask{18}='on';p_mask{19}='on';
      |     case 'Drive train data for 1 wind turbine'
      |         p_mask{20}='on';p_mask{21}='on';p_mask{22}='on';p_mask{23}='on';
      |         p_mask{24}='on';
      |     case 'Control parameters for 1 wind turbine'
      |         p_mask{25}='on';p_mask{26}='on';p_mask{27}='on';
      |         p_mask{28}='on';p_mask{29}='on';p_mask{30}='on';p_mask{31}='on';
      |         p_mask{32}='on';p_mask{33}='on';p_mask{34}='on';p_mask{35}='on';
      | end
      | 
      | ParVisible={'on','on',p_mask{3},p_mask{4},p_mask{5},p_mask{6},...
      |     p_mask{7},p_mask{8},p_mask{9},p_mask{10},p_mask{11},p_mask{12},...
      |     p_mask{13},p_mask{14},p_mask{15},p_mask{16},p_mask{17},p_mask{18},...
      |     p_mask{19},p_mask{20},p_mask{21},p_mask{22},p_mask{23},p_mask{24},...
      |     p_mask{25},p_mask{26},p_mask{27},p_mask{28},p_mask{29},p_mask{30},...
      |     p_mask{31},p_mask{32},p_mask{33},p_mask{34},p_mask{35},'on'};
      | %
      | set_param(BlockName,'MaskVisibilities',ParVisible);
      | set_param(BlockName,'DisplayTurbChar',Param_DisplayTurbChar);
      mask Display: disp(' ');
  Wind Farm Scope : Scope  NumInputPorts=6
  A : PMIOPort  Side=Left
  B : PMIOPort  Port=2  Side=Left
  C : PMIOPort  Port=3  Side=Left
  wires:
  Constant1/1 -> Wind Farm/2(Qref_pu)
  [Vabc_B2] -> Wind Farm Scope/1  "Vabc_B575 (pu)"
  Demux/1 -> Wind Farm Scope/5  "P (MW)"
  Bus Selector/1 -> Wind Farm Scope/3  "<Vdc_V>"
  Demux/2 -> Wind Farm Scope/6  "Q (Mvar)"
  Mux/1 -> MW/1
  Bus Selector/2 -> Wind Farm Scope/4  "<wr_pu>"
  Wind Farm/1(m) -> Bus Selector/1
  Bus Selector/3 -> Mux/1  "<P_pu>"
  Bus Selector/4 -> Mux/2  "<Q_pu>"
  MW/1 -> Demux/1
  [Iabc_B2] -> Wind Farm Scope/2  "Iabc_B575 (pu)"
  Constant/1 -> Wind Farm/1("Wind (m/s) ")
  connections:
  B2 (690 V)/LConn2 -- 34.5 kV/ 690V 5*2.5 MVA/RConn2
  B2 (690 V)/RConn1 -- Wind Farm/LConn1
  B2 (690 V)/LConn1 -- 34.5 kV/ 690V 5*2.5 MVA/RConn1
  B2 (690 V)/LConn3 -- 34.5 kV/ 690V 5*2.5 MVA/RConn3
  B2 (690 V)/RConn3 -- Wind Farm/LConn3
  Wind Farm/LConn2 -- B2 (690 V)/RConn2
  34.5 kV/ 690V 5*2.5 MVA/LConn2 -- 5 km line/RConn2
  5 km line/LConn1 -- 230 kV/34.5 kV 47 MVA/RConn1
  A/RConn1 -- 230 kV/34.5 kV 47 MVA/LConn1
  5 km line/LConn3 -- 230 kV/34.5 kV 47 MVA/RConn3
  34.5 kV/ 690V 5*2.5 MVA/LConn1 -- 5 km line/RConn1
  34.5 kV/ 690V 5*2.5 MVA/LConn3 -- 5 km line/RConn3
  5 km line/LConn2 -- 230 kV/34.5 kV 47 MVA/RConn2
  230 kV/34.5 kV 47 MVA/LConn2 -- B/RConn1
  230 kV/34.5 kV 47 MVA/LConn3 -- C/RConn1

== system WindFarmType4AverageModel/More Info ==

== system WindFarmType4AverageModel/Noble Altona (97.5 MW) ==
  230 kV/34.5 kV 47 MVA : spsThreePhaseTransformerTwoWindingsLib/Three-Phase Transformer (Two Windings)  Winding1Connection=Yg  Winding2Connection=Delta (D1)  CoreType=Three single-phase transformers  SetSaturation=off  Hysteresis=off  DataFile='basic_model'  SetInitialFlux=off  Measurements=None  UNITS=pu  NominalPower=[47e6 60 ]  Winding1="[ 230e3  0.08/30   0.08 ]"  Winding2="[34.5e3  0.08/30  0.08]"  Rm=500  Lm=500  L0=0.5  Saturation="[ 0,0  ;  0.005,1.2  ;  1.0,1.4 ]"  InitialFluxes=[ 0.8 , -0.8 , 0.7 ]  BreakLoop=off  DiscreteSolver=Trapezoidal iterative  DataType=off  TransfoNumber=0
  34.5 kV/ 690V 5*2.5 MVA : spsThreePhaseTransformerTwoWindingsLib/Three-Phase Transformer (Two Windings)  Winding1Connection=Delta (D11)  Winding2Connection=Yg  CoreType=Three single-phase transformers  SetSaturation=off  Hysteresis=off  DataFile='hysteresis'  SetInitialFlux=off  Measurements=None  UNITS=pu  NominalPower="[2.5e6*5  60]"  Winding1=[34.5e3 , 0.025/30 , 0.025]  Winding2=[690, 0.025/30 , 0.025]  Rm=500  Lm=inf  L0=0.5  Saturation=[ 0,0 ; 0.0024,1.2 ; 1.0,1.52 ]  InitialFluxes=[ 0.8 , -0.8 , 0.7 ]  BreakLoop=off  DiscreteSolver=Trapezoidal iterative  DataType=off  TransfoNumber=0
  5 km line : spsThreePhasePISectionLineLib/Three-Phase PI Section Line  LConnTagsString=a|b|c  RConnTagsString=A|B|C  Length=5  Frequency=60  Resistances=[0.1153 0.413]  Inductances=[1.05e-3 3.32e-3]  Capacitances=[11.33e-009 5.01e-009]
  B3 (690 V) : spsThreePhaseVIMeasurementLib/Three-Phase V-I Measurement  VoltageMeasurement=phase-to-ground  SetLabelV=on  LabelV=Vabc_B3  Vpu=on  VpuLL=off  CurrentMeasurement=yes  SetLabelI=on  LabelI=Iabc_B3  Ipu=on  Pbase=5*2e6/0.9  Vbase=690  OutputType=Complex  PhasorSimulation=off  PSBequivalent=0
  Bus Selector : BusSelector  OutputSignals=Vdc_V,wr_pu,PQ_pu.P_pu,PQ_pu.Q_pu
  Constant : Constant  Value=15
  Constant1 : Constant  Value=0
  Demux : Demux  Outputs=2
  MW : Gain  Gain=65*1.5/0.9  SaturateOnIntegerOverflow=on  OutDataTypeStr=Inherit: Same as input  ParamDataTypeStr=Inherit: Same as input
  Mux : Mux  Inputs=2
  Wind Farm : Subsystem  LoadFcn=%find_system(gcs,'FollowLinks', 'on', 'LookUnderMasks', 'all');  mask(Wind Turbine: Model 7){Nb_wt=65, ShowParameters=Generator data for 1 wind turbine, nom=[1.5e6/0.9 690 60], Reactances=[ 1.305, 0.296, 0.252, 0.474,  0.243,  0.18 ], Time_constants=[  4.49  0.0681  0.0513  ], Resistance=0.006, mec=[0.62 0.01 1], init=[ 0  0  0  0  0  0  0  0  1 ], Vnom=575, Imax_grid_conv=1.1, RL_grid=[ 0.15 0.15/50], C_var_filter1=150e3, Vdc_nom=1100, C_DClink1=90000e-6, L_R_Boost=[0.0012     5e-3], Pmec1=2e6, wind_speed_CpMax=11, wind0=11, DisplayTurbChar=off, H_WT=4.32, Ksh=0.3, D_mutual=1.5, w_wt0=1, torque0=1, Kdc=[1.1   27.5], Ki_var_reg=0.05, Ki_volt_reg=2, Kgrid_side_cur_reg=[1  50], Kspeed=[5 1], Kboost_cur_reg=[0.025 100], Kp_pitch=15, Kcompensation=[1.5  6], Kfield=[10  20], pitch_max=27, pitch_rate=10, Ts=Ts}
      mask prompts: Nb_wt "Number of wind turbines:"; ShowParameters "Display:"; nom "Nom. power, L-L volt. and freq.: [Pn (VA), Vn (Vrms), fn (Hz)]"; Reactances "Reactances [Xd Xd' Xd'' Xq Xq'' Xl] (p.u.):"; Time_constants "Time constants [Tdo' Tdo'' Tq''] (s):"; Resistance "Resistance Rs (p.u.):"; mec "Inertia constant, friction factor, and pairs of poles: [ H(s)  F(p.u.)  p ]"; init "Initial conditions: [dw(%) th(deg) ia,ib,ic(pu) pha,phb,phc(deg) Vf(pu)]:"; Vnom "Grid-side converter nominal AC voltage (V):"; Imax_grid_conv "Grid-side converter maximum AC current (pu based on generator power and converter nominal AC voltage):"; RL_grid "Grid-side coupling inductor [ L(pu) R(pu),pu based on generator power and converter nominal AC voltage] :"; C_var_filter1 "Line filter capacitor (Q=50) (var):"; Vdc_nom "Nominal DC bus voltage (V)"; C_DClink1 "DC bus capacitor (F):"; L_R_Boost "Boost converter inductance [L(H) R(ohm)]:"; Pmec1 "Nominal mechanical output power (W):"; wind_speed_CpMax "Wind speed at nominal speed and at Cp max (must be between 6 m/s and 30 m/s) (m/s):"; wind0 "Initial wind speed (m/s):"; DisplayTurbChar "Display wind turbine power characteristics:"; H_WT "Wind turbine inertia constant H (s):"; Ksh "Shaft spring constant refer to high-speed shaft (pu of nominal mechanical torque/rad):"; D_mutual "Shaft mutual damping (pu of nominal mechanical torque/pu dw):"; w_wt0 "Turbine initial speed (pu of nominal speed):"; torque0 "Initial output torque (pu of nominal mechanical torque):"; Kdc "DC bus voltage regulator gains [Kp Ki]:"; Ki_var_reg "Grid-side converter var regulator gain [ Ki]:"; Ki_volt_reg "Grid-side converter voltage regulator gain [ Ki]:"; Kgrid_side_cur_reg "Grid-side converter current regulator gains [Kp Ki]:"; Kspeed "Speed regulator gains [Kp Ki]:"; Kboost_cur_reg "Boost inductor current regulator gains [Kp Ki]:"; Kp_pitch "Pitch controller gain [Kp]:"; Kcompensation "Pitch compensation gains [Kp Ki]:"; Kfield "Field excitation gains [Kp Ki]:"; pitch_max "Maximum pitch angle (deg):"; pitch_rate "Maximum rate of change of pitch angle (deg/s)"; Ts "Sample time (s):"
      mask help: This block implements a model of a variable speed pitch controlled wind turbine using a synchronous generator.
      mask init: same as WindFarmType4AverageModel/Jericho Rise (77.7 MW)/Wind Farm
      mask TypeOptions ShowParameters: Generator data for 1 wind turbine | Converters data for 1 wind turbine | Turbine data for 1 wind turbine | Drive train data for 1 wind turbine | Control parameters for 1 wind turbine
      mask Callback ShowParameters:
      | BlockName=getfullname(gcb);
      | %
      | Param_Show=get_param(BlockName,'ShowParameters');
      | Param_DisplayTurbChar=get_param(BlockName,'DisplayTurbChar');
      | 
      | p_mask{3}='off';p_mask{4}='off';p_mask{5}='off';
      | p_mask{6}='off';p_mask{7}='off';p_mask{8}='off';p_mask{9}='off';
      | p_mask{10}='off';p_mask{11}='off';p_mask{12}='off';p_mask{13}='off';
      | p_mask{14}='off';p_mask{15}='off';p_mask{16}='off';p_mask{17}='off';
      | p_mask{18}='off';p_mask{19}='off';p_mask{20}='off';p_mask{21}='off';
      | p_mask{22}='off';p_mask{23}='off';p_mask{24}='off';p_mask{25}='off';
      | p_mask{26}='off';p_mask{27}='off';p_mask{28}='off';p_mask{29}='off';
      | p_mask{30}='off';p_mask{31}='off';p_mask{32}='off';p_mask{33}='off';
      | p_mask{34}='off';p_mask{35}='off';
      | 
      | switch Param_Show
      | 	case 'Generator data for 1 wind turbine'
      | 		p_mask{3}='on';p_mask{4}='on';p_mask{5}='on';
      |         p_mask{6}='on';p_mask{7}='on';p_mask{8}='on';
      |     case 'Converters data for 1 wind turbine'
      | 		p_mask{9}='on';p_mask{10}='on';p_mask{11}='on';
      |         p_mask{12}='on';p_mask{13}='on';p_mask{14}='on';p_mask{15}='on';
      | 	case 'Turbine data for 1 wind turbine'
      | 		p_mask{16}='on';p_mask{17}='on';p_mask{18}='on';p_mask{19}='on';
      |     case 'Drive train data for 1 wind turbine'
      |         p_mask{20}='on';p_mask{21}='on';p_mask{22}='on';p_mask{23}='on';
      |         p_mask{24}='on';
      |     case 'Control parameters for 1 wind turbine'
      |         p_mask{25}='on';p_mask{26}='on';p_mask{27}='on';
      |         p_mask{28}='on';p_mask{29}='on';p_mask{30}='on';p_mask{31}='on';
      |         p_mask{32}='on';p_mask{33}='on';p_mask{34}='on';p_mask{35}='on';
      | end
      | 
      | ParVisible={'on','on',p_mask{3},p_mask{4},p_mask{5},p_mask{6},...
      |     p_mask{7},p_mask{8},p_mask{9},p_mask{10},p_mask{11},p_mask{12},...
      |     p_mask{13},p_mask{14},p_mask{15},p_mask{16},p_mask{17},p_mask{18},...
      |     p_mask{19},p_mask{20},p_mask{21},p_mask{22},p_mask{23},p_mask{24},...
      |     p_mask{25},p_mask{26},p_mask{27},p_mask{28},p_mask{29},p_mask{30},...
      |     p_mask{31},p_mask{32},p_mask{33},p_mask{34},p_mask{35},'on'};
      | %
      | set_param(BlockName,'MaskVisibilities',ParVisible);
      | set_param(BlockName,'DisplayTurbChar',Param_DisplayTurbChar);
      mask Display: disp(' ');
  Wind Farm Scope : Scope  NumInputPorts=6
  A : PMIOPort  Side=Left
  B : PMIOPort  Port=2  Side=Left
  C : PMIOPort  Port=3  Side=Left
  wires:
  Constant1/1 -> Wind Farm/2(Qref_pu)
  [Vabc_B3] -> Wind Farm Scope/1  "Vabc_B575 (pu)"
  Demux/1 -> Wind Farm Scope/5  "P (MW)"
  Bus Selector/1 -> Wind Farm Scope/3  "<Vdc_V>"
  Demux/2 -> Wind Farm Scope/6  "Q (Mvar)"
  Mux/1 -> MW/1
  Bus Selector/2 -> Wind Farm Scope/4  "<wr_pu>"
  Wind Farm/1(m) -> Bus Selector/1
  Bus Selector/3 -> Mux/1  "<P_pu>"
  Bus Selector/4 -> Mux/2  "<Q_pu>"
  MW/1 -> Demux/1
  [Iabc_B3] -> Wind Farm Scope/2  "Iabc_B575 (pu)"
  Constant/1 -> Wind Farm/1("Wind (m/s) ")
  connections:
  B3 (690 V)/LConn2 -- 34.5 kV/ 690V 5*2.5 MVA/RConn2
  B3 (690 V)/RConn1 -- Wind Farm/LConn1
  B3 (690 V)/LConn1 -- 34.5 kV/ 690V 5*2.5 MVA/RConn1
  B3 (690 V)/LConn3 -- 34.5 kV/ 690V 5*2.5 MVA/RConn3
  B3 (690 V)/RConn3 -- Wind Farm/LConn3
  Wind Farm/LConn2 -- B3 (690 V)/RConn2
  34.5 kV/ 690V 5*2.5 MVA/LConn2 -- 5 km line/RConn2
  5 km line/LConn1 -- 230 kV/34.5 kV 47 MVA/RConn1
  C/RConn1 -- 230 kV/34.5 kV 47 MVA/LConn3
  A/RConn1 -- 230 kV/34.5 kV 47 MVA/LConn1
  5 km line/LConn3 -- 230 kV/34.5 kV 47 MVA/RConn3
  34.5 kV/ 690V 5*2.5 MVA/LConn1 -- 5 km line/RConn1
  34.5 kV/ 690V 5*2.5 MVA/LConn3 -- 5 km line/RConn3
  B/RConn1 -- 230 kV/34.5 kV 47 MVA/LConn2
  5 km line/LConn2 -- 230 kV/34.5 kV 47 MVA/RConn2
